simulink model "Cruise_control"  (R2021a)
settings: Solver=VariableStepAuto  StartTime=0.0  StopTime=10.0  RelTol=1e-3
values from neighbouring files (symbols this model uses):
  b = 50.0    [week2_prob3.sldd]
  m = 1000.0    [week2_prob3.sldd]
settings Model: DataDictionary=week2_prob3.sldd  Creator=varunraj  LastModifiedBy=varunraj
settings DataIOCC: SaveOutput=off  SaveTime=off

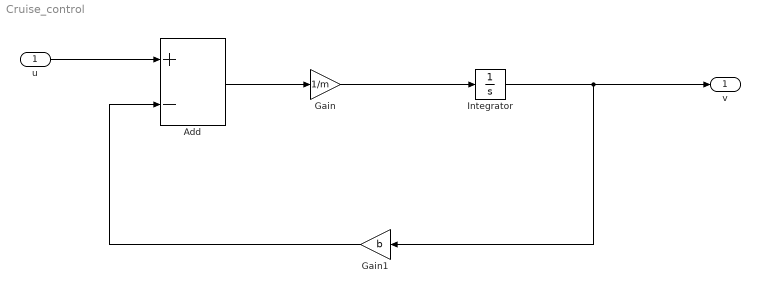
== system Cruise_control ==
  u : Inport  OutDataTypeStr=double  PortDimensions=1
  Add : Sum  Inputs=+-
  Gain : Gain  Gain=1/m
  Gain1 : Gain  Gain=b
  Integrator : Integrator
  v : Outport  OutDataTypeStr=double  PortDimensions=1  SampleTime=0
  wires:
  Gain1/1 -> Add/2
  Add/1 -> Gain/1
  Integrator/1 -> Gain1/1, v/1
  Gain/1 -> Integrator/1
  u/1 -> Add/1
